simulink library "AdvancedMux"  (R2014b)
settings: Solver=ode45  StartTime=0.0  StopTime=10.0  RelTol=1e-3
settings Model: Creator=Hp  LastModifiedBy=Hp

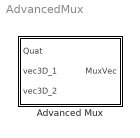
== system AdvancedMux ==
  Advanced Mux : Subsystem

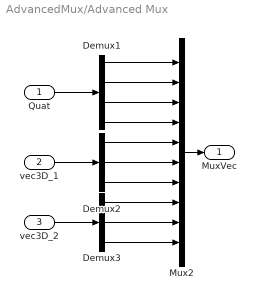
== system AdvancedMux/Advanced Mux ==
  Quat : Inport
  vec3D_1 : Inport  Port=2
  vec3D_2 : Inport  Port=3
  Demux1 : Demux
  Demux2 : Demux  Outputs=3
  Demux3 : Demux  Outputs=3
  Mux2 : Mux  Inputs=10
  MuxVec : Outport
  wires:
  Mux2/1 -> MuxVec/1
  Demux3/3 -> Mux2/10
  Demux2/2 -> Mux2/6
  Demux1/4 -> Mux2/4
  Demux3/1 -> Mux2/8
  Demux2/1 -> Mux2/5
  vec3D_2/1 -> Demux3/1
  Demux2/3 -> Mux2/7
  Demux3/2 -> Mux2/9
  Quat/1 -> Demux1/1
  Demux1/3 -> Mux2/3
  Demux1/2 -> Mux2/2
  vec3D_1/1 -> Demux2/1
  Demux1/1 -> Mux2/1
